simulink model "bilinearfilt"  (R2020b)
settings: Solver=VariableStepAuto  StartTime=0.0  StopTime=10.0  MaxStep=0.01  RelTol=1e-3
settings Model: Creator=shivanshu shukla  LastModifiedBy=shivanshu shukla

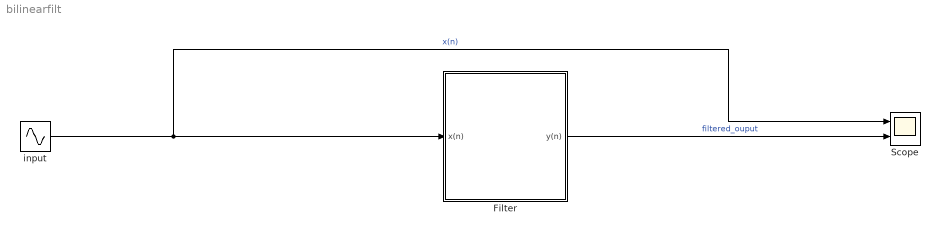
== system bilinearfilt ==
  Filter : Subsystem
  Scope : Scope  NumInputPorts=2
  input : Sin  Amplitude=5  Frequency=2*pi*100  SampleTime=0.0002
  wires:
  input/1 -> Scope/1, Filter/1(x(n))  "x(n)"
  Filter/1(y(n)) -> Scope/2  "filtered_ouput"

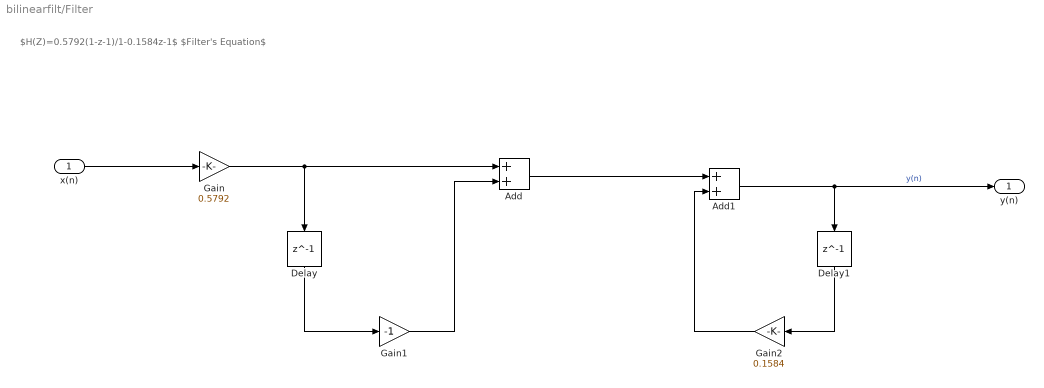
== system bilinearfilt/Filter ==
  note: $H(Z)=0.5792(1-z-1)/1-0.1584z-1$ $Filter's Equation$
  x(n) : Inport
  Add : Sum
  Add1 : Sum
  Delay : Delay  DelayLength=1
  Delay1 : Delay  DelayLength=1
  Gain : Gain  Gain=0.5792
  Gain1 : Gain  Gain=-1
  Gain2 : Gain  Gain=0.1584
  y(n) : Outport
  wires:
  Gain2/1 -> Add1/2
  Delay/1 -> Gain1/1
  Gain/1 -> Add/1, Delay/1
  Delay1/1 -> Gain2/1
  Gain1/1 -> Add/2
  Add1/1 -> y(n)/1, Delay1/1  "y(n)"
  Add/1 -> Add1/1
  x(n)/1 -> Gain/1
